simulink model "EXAMPLE_DecodeMavlink_blocks"  (R2019b)
settings: Solver=FixedStepAuto  StartTime=0.0  StopTime=inf  FixedStep=0.01  RelTol=1e-3  EnableMultiTasking=on
undefined symbols (not defined in the file): serial
libraries: etargetslib x4, instrumentlib x2
settings Model: SimulationMode=external  ExtModeTrigDuration=10  Creator=cuencaa  LastModifiedBy=andrei
settings SolverCC: PositivePriorityOrder=on
settings DataIOCC: ReturnWorkspaceOutputs=off
settings OptimizationCC: EnhancedBackFolding=on  PassReuseOutputArgsAs=Individual arguments  MaxStackSize=64  OptimizeBlockOrder=speed  DifferentSizesBufferReuse=on  OptimizationCustomize=off  EfficientTunableParamExpr=on
settings DebuggingCC: ParameterTunabilityLossMsg=error  PregeneratedLibrarySubsystemCodeDiagnostic=none  ArithmeticOperatorsInVariantConditions=warning
settings HardwareCC: ProdBitPerPointer=32  ProdBitPerSizeT=32  ProdBitPerPtrDiffT=32  ProdLargestAtomicInteger=Long  ProdLargestAtomicFloat=Double  ProdWordSize=32  ProdLongLongMode=on  ProdHWDeviceType=ARM Compatible->ARM Cortex
settings SFSimCC: SimUseLocalCustomCode=off  MATLABDynamicMemAlloc=off  CustomCodeUndefinedFunction=UseInterfaceOnly
settings RTWCC: SystemTargetFile=ert.tlc  HardwareBoard=PX4 Pixhawk 1  TLCOptions="-aInlineSetEventsForThisBaseRateFcn=TLC_FALSE -aSuppressMultiTaskScheduler=TLC_FALSE  -aRateBasedStepFcn=0"  TemplateMakefile=ert_default_tmf  GenerateReport=on  RTWUseLocalCustomCode=off  Toolchain=GNU Tools for PX4 Autopilots  IncludeHyperlinkInReport=on  LaunchReport=on  TargetLang=C++  GenerateTraceInfo=on  GenerateTraceReport=on  GenerateTraceReportSl=on  GenerateTraceReportSf=on  GenerateTraceReportEml=on
settings CodeAppCC: ForceParamTrailComments=on  IgnoreCustomStorageClasses=off  OperatorAnnotations=on  SimulinkDataObjDesc=on  SFDataObjDesc=on  InsertBlockDesc=on

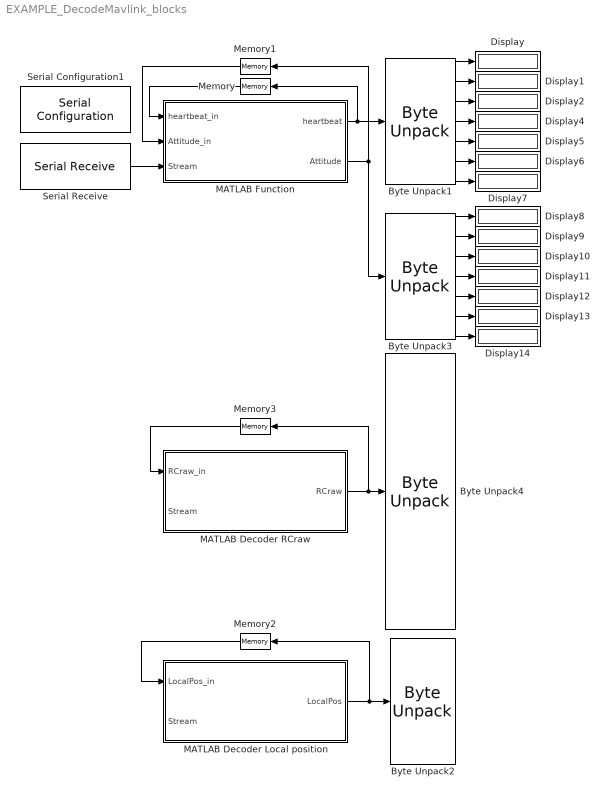
== system EXAMPLE_DecodeMavlink_blocks ==
  Byte Unpack1 : etargetslib/Byte Unpack  dimensions={[1],[1],[1],[1],[1],[1],[1]}  datatypes={'uint32','uint8','uint8','uint8','uint8','uint8','uint8'}  byteAlign=1
      settings: SourceProductName=MATLAB Coder
  Byte Unpack2 : etargetslib/Byte Unpack  dimensions={[1],[1],[1],[1],[1],[1],[1]}  datatypes={'uint32','single','single','single','single','single','single'}  byteAlign=1
      settings: SourceProductName=MATLAB Coder
  Byte Unpack3 : etargetslib/Byte Unpack  dimensions={[1],[1],[1],[1],[1],[1],[1]}  datatypes={'uint32','single','single','single','single','single','single'}  byteAlign=1
      settings: SourceProductName=MATLAB Coder
  Byte Unpack4 : etargetslib/Byte Unpack  dimensions={[1],[1],[1],[1],[1],[1],[1],[1],[1],[1],[1]}  datatypes={'uint32','uint16','uint16','uint16','uint16','uint16','uint16','uint16','uint16','uint8','uint8'}  byteAlign=1
      settings: SourceProductName=MATLAB Coder
  Display{,1..2,4..14} (14 alike) : Display
  MATLAB Decoder Local position : MATLAB Function  TreatAsAtomicUnit=on
  MATLAB Decoder RCraw : MATLAB Function  TreatAsAtomicUnit=on
  MATLAB Function : MATLAB Function  TreatAsAtomicUnit=on
  Memory : Memory  InitialCondition=uint8(zeros(9,1));
  Memory1 : Memory  InitialCondition=uint8(zeros(28,1))
  Memory2 : Memory  InitialCondition=uint8(zeros(28,1))
  Memory3 : Memory  InitialCondition=uint8(zeros(22,1));
  Serial Configuration1 : instrumentlib/Serial Configuration  Priority=-200000  ComPortMenu=<Please select a port...>  ComPort=COM12  ObjConstructor=serial('COM12');  BaudRate=57600  DataBits=8  Parity=none  StopBits=1  FlowControl=none  Timeout=10  ByteOrder=LittleEndian
  Serial Receive : instrumentlib/Serial Receive  ComPortMenu=<Please select a port...>  ComPort=COM12  ObjConstructor=serial('COM12');  Terminator=<none>  DataSize=263  DataType=uint8  EnableBlockingMode=on  ActionDataUnavailable=Output last received value  CustomValue=0  SampleTime=0.01
  wires:
  MATLAB Function/1(heartbeat) -> Byte Unpack1/1, Memory/1
  MATLAB Function/2(Attitude) -> Byte Unpack3/1, Memory1/1
  Memory/1 -> MATLAB Function/1(heartbeat_in)
  Memory1/1 -> MATLAB Function/2(Attitude_in)
  Serial Receive/1 -> MATLAB Function/3(Stream)
  Byte Unpack1/1 -> Display/1
  Byte Unpack1/2 -> Display1/1
  Byte Unpack1/3 -> Display2/1
  Byte Unpack1/4 -> Display4/1
  Byte Unpack1/5 -> Display5/1
  Byte Unpack1/6 -> Display6/1
  Byte Unpack1/7 -> Display7/1
  Byte Unpack3/7 -> Display14/1
  Byte Unpack3/1 -> Display8/1
  Byte Unpack3/2 -> Display9/1
  Byte Unpack3/3 -> Display10/1
  Byte Unpack3/4 -> Display11/1
  Byte Unpack3/5 -> Display12/1
  Byte Unpack3/6 -> Display13/1
  MATLAB Decoder RCraw/1(RCraw) -> Memory3/1, Byte Unpack4/1
  Memory3/1 -> MATLAB Decoder RCraw/1(RCraw_in)
  MATLAB Decoder Local position/1(LocalPos) -> Memory2/1, Byte Unpack2/1
  Memory2/1 -> MATLAB Decoder Local position/1(LocalPos_in)

== matlab function EXAMPLE_DecodeMavlink_blocks/MATLAB Function ==
  data: heartbeat_in input; Attitude_in input; Stream input; heartbeat output uint8; Attitude output uint8
function [heartbeat,Attitude] = MavlinkDecoder(heartbeat_in,Attitude_in,Stream)
%% CODE DEVELOPED BY ANDREI CUENCA
%EMBRY RIDDLE Aeronautical university
%Advance Dynamics and Control Laboratory
%Version 1 - Jun 2019


% The following block Decodes the specified Mav packages listed in Outputs. 
% The input for this function is the stream received from the serial 
% comunication and the values from the last sample time. 

%% Initial definitions ----------------------------------------------------
SM=0;       %Flag Start byte Detected
a=1;        %Count for bytes
FHB=0;      %Flag HeartBeat Msg Saved
FATT=0;     %Flag Attitude Msg Daved

Size=length(Stream);

% This secction is define to hold the last value if a new value was not
% detected in the package
heartbeat=heartbeat_in;
Attitude=Attitude_in;

%Defines CRC conditions and generator--------------
%The CRC is used to check the package integrity. If data is corrupted 
%it will be discarted keeping last value known given by the inputs.
CRC_HB=uint8(50);   %CRC_Extra value for Heartbeat
CRC_ATT=uint8(39);  %CRC_Extra value for Attitude
CRC_def=comm.CRCGenerator('z^16 + z^12 + z^5 + 1','DirectMethod',true,...
    'InitialConditions',[1 1 1 1 1 1 1 1 1 1 1 1 1 1 1 1],...
    'ReflectInputBytes',true,'ReflectChecksums',true);
            
%% Decode process ---------------------------------------------------------
while a<230
    if (SM==0 && Stream(a)==254)

        %Tells if a message is being read
        SM=1;
        %Read header ID 0xFE (254) if detected
        PL=Stream(a+1);     %Read Payload
        SysID=Stream(a+3);  %Read System ID
        CompID=Stream(a+4); %Read ComponentID
        ID=Stream(a+5);     %Read Message ID
        
        % Decode heartbeat-------------------------------------------------
        if (SM== 1 && ID==0 && PL==9 && FHB==0)
            
            %Reads the Package and adds the CRC_extra
            PKG=[Stream(a+1:a+14)' CRC_HB];
            
            %Extract CRC bytes from incoming MSG 
            CRC1_R=Stream(a+15);
            CRC2_R=Stream(a+16);
            
            %Convert Package in binary stream
            PKG=de2bi(PKG,8,'left-msb');
            
            %Prealocatting binary Stream
            PKG_bin=zeros(1,15*8);
            PKG_bin(1:8)=PKG(1,:);
            for b=2:15
                PKG_bin(b*8-7:b*8)= PKG(b,:);
            end
            
            %Calculates CRC with received Package
            CRC=CRC_def(logical(PKG_bin'));
            
            CRC=CRC';
            CRC2_C=bi2de(CRC(end-15:end-8),'left-msb');
            CRC1_C=bi2de(CRC(end-7:end),'left-msb');
            
            %Compares CRC received with Calculated for MSG integrity
            if (CRC1_R==CRC1_C && CRC2_R==CRC2_C)
                heartbeat=Stream(a+6:a+14);
                SM=0;
                FHB=1;
            else
                SM=0;
                a=a+1;
            end
            
            
        %Case Attitude----------------------------------------------------    
        elseif (SM==1 && ID==30 && PL==28 && FATT==0)
            
            PKG=[Stream(a+1:a+33)' CRC_ATT];    
            %Check integrity of package extrackting CRC bytes 
            CRC1_R=Stream(a+34);
            CRC2_R=Stream(a+35);
            
            %Convert Package in binary stream
            PKG=de2bi(PKG,8,'left-msb');
            
            %Preallocating binary Stream
            PKG_bin=zeros(1,34*8);
            PKG_bin(1:8)=PKG(1,:);
            for b=2:34
                PKG_bin(b*8-7:b*8)= PKG(b,:);
            end
            
            %Calculates CRC with received Package
            CRC=CRC_def(logical(PKG_bin'));
            
            CRC=CRC';
            CRC2_C=bi2de(CRC(end-15:end-8),'left-msb');
            CRC1_C=bi2de(CRC(end-7:end),'left-msb');
            
            %Compares CRC received with Calculated for MSG integrity
            if (CRC1_R==CRC1_C && CRC2_R==CRC2_C)
                Attitude=Stream(a+6:a+33);
                SM=0;
                FATT=1;
            else
                SM=0;
                a=a+1;
            end
        
        else
            SM=0;
            a=a+1;
        end
     else
         a=a+1;
         SM=0;
     end
    % If both messages were found stops the loop
     if FHB==1 && FATT==1
         break
     end
    
end
 
 
end

== matlab function EXAMPLE_DecodeMavlink_blocks/MATLAB Decoder Local position ==
  data: LocalPos_in input; Stream input; LocalPos output uint8
function LocalPos   = MavlinkDecoder(LocalPos_in,Stream)
%% CODE DEVELOPED BY ANDREI CUENCA
%EMBRY RIDDLE Aeronautical university
%Advance Dynamics and Control Laboratory
%Version 1 - Jun 2019


% The following block Decodes the specified Mav packages listed in Outputs. 
% The input for this function is the stream received from the serial 
% comunication and the values from the last sample time. 

%% Initial definitions ----------------------------------------------------
SM=0;       %Flag Start byte Detected
a=1;        %Count for bytes
FLP=0;      %Flag HeartBeat Msg Saved

% This secction is defined to hold the last value if a new value was not
% detected in the package
LocalPos=LocalPos_in;

%Defines CRC conditions and generator--------------
%The CRC is used to check the package integrity. If data is corrupted 
%it will be discarted keeping last value known given by the inputs.

CRC_LP=uint8(185); 
CRC_def=comm.CRCGenerator('z^16 + z^12 + z^5 + 1','DirectMethod',true,...
    'InitialConditions',[1 1 1 1 1 1 1 1 1 1 1 1 1 1 1 1],...
    'ReflectInputBytes',true,'ReflectChecksums',true);
            
%% Decode process ---------------------------------------------------------
while a<150
    if (SM==0 && Stream(a)==254)

        %Tells if a message is being read
        SM=1;
        %Read header ID 0xFE (254) if detected
        PL=Stream(a+1);     %Read Payload
        SysID=Stream(a+3);  %Read System ID
        CompID=Stream(a+4); %Read ComponentID
        ID=Stream(a+5);     %Read Message ID
        
        %Case Attitude----------------------------------------------------    
        if (SM==1 && ID==32 && PL==28 && FLP==0)
            
            PKG=[Stream(a+1:a+33)' CRC_LP];    
            %Check integrity of package extrackting CRC bytes 
            CRC1_R=Stream(a+34);
            CRC2_R=Stream(a+35);
            
            %Convert Package in binary stream
            PKG=de2bi(PKG,8,'left-msb');
            
            %Preallocating binary Stream
            PKG_bin=zeros(1,34*8);
            PKG_bin(1:8)=PKG(1,:);
            for b=2:34
                PKG_bin(b*8-7:b*8)= PKG(b,:);
            end
            
            %Calculates CRC with received Package
            CRC=CRC_def(logical(PKG_bin'));
            
            CRC=CRC';
            CRC2_C=bi2de(CRC(end-15:end-8),'left-msb');
            CRC1_C=bi2de(CRC(end-7:end),'left-msb');
            
            %Compares CRC received with Calculated for MSG integrity
            if (CRC1_R==CRC1_C && CRC2_R==CRC2_C)
                LocalPos=Stream(a+6:a+33);
                SM=0;
                FLP=1;
            else
                SM=0;
                a=a+1;
            end
        
        else
            SM=0;
            a=a+1;
        end
     else
         a=a+1;
         SM=0;
     end
    % If both messages were found stops the loop
     if FLP==1
         break
     end
    
end
 
 
end

== matlab function EXAMPLE_DecodeMavlink_blocks/MATLAB Decoder RCraw ==
  data: RCraw_in input; Stream input; RCraw output uint8
function RCraw    = MavlinkDecoder(RCraw_in,Stream)
%% CODE DEVELOPED BY ANDREI CUENCA
%EMBRY RIDDLE Aeronautical university
%Advance Dynamics and Control Laboratory
%Version 1 - Jun 2019


% The following block Decodes the specified Mav packages listed in Outputs. 
% The input for this function is the stream received from the serial 
% comunication and the values from the last sample time. 

%% Initial definitions ----------------------------------------------------
SM=0;       %Flag Start byte Detected
a=1;        %Count for bytes
FRCR=0;      %Flag  Msg Saved


% This secction is define to hold the last value if a new value was not
% detected in the package
RCraw=RCraw_in;


%Defines CRC conditions and generator--------------
%The CRC is used to check the package integrity. If data is corrupted 
%it will be discarted keeping last value known given by the inputs.
CRC_RCR=uint8(244);   %CRC_Extra value for Heartbeat
CRC_def=comm.CRCGenerator('z^16 + z^12 + z^5 + 1','DirectMethod',true,...
    'InitialConditions',[1 1 1 1 1 1 1 1 1 1 1 1 1 1 1 1],...
    'ReflectInputBytes',true,'ReflectChecksums',true);
            
%% Decode process ---------------------------------------------------------
while a<230
    if (SM==0 && Stream(a)==254)
        
        %Tells if a message is being read
        SM=1;
        %Read header ID 0xFE (254) if detected
        PL=Stream(a+1);     %Read Payload
        SysID=Stream(a+3);  %Read System ID
        CompID=Stream(a+4); %Read ComponentID
        ID=Stream(a+5);     %Read Message ID
        
        % Decode heartbeat-------------------------------------------------
        if (SM== 1 && ID==35 && PL==22 && FRCR==0)
            
            %Reads the Package and adds the CRC_extra
            PKG=[Stream(a+1:a+27)' CRC_RCR];
            
            %Extract CRC bytes from incoming MSG 
            CRC1_R=Stream(a+28);
            CRC2_R=Stream(a+29);
            
            %Convert Package in binary stream
            PKG=de2bi(PKG,8,'left-msb');
            
            %Prealocatting binary Stream
            PKG_bin=zeros(1,28*8);
            PKG_bin(1:8)=PKG(1,:);
            for b=2:28
                PKG_bin(b*8-7:b*8)= PKG(b,:);
            end
            
            %Calculates CRC with received Package
            CRC=CRC_def(logical(PKG_bin'));
            
            CRC=CRC';
            CRC2_C=bi2de(CRC(end-15:end-8),'left-msb');
            CRC1_C=bi2de(CRC(end-7:end),'left-msb');
            
            %Compares CRC received with Calculated for MSG integrity
            if (CRC1_R==CRC1_C && CRC2_R==CRC2_C)
                RCraw=Stream(a+6:a+27);
                SM=0;
                FRCR=1;
            else
                SM=0;
                a=a+1;
            end
            
            
        
        else
            SM=0;
            a=a+1;
        end
     else
         a=a+1;
         SM=0;
     end
    % If both messages were found stops the loop
     if FRCR==1
         break
     end
    
end
 
 
end
